simulink model "Solver_simulink"  (R2026a)
settings: Solver=VariableStepAuto  StopTime=5  RelTol=1e-4
values from neighbouring files (symbols this model uses):
  a = 0.01    [MassSpringDamper.m]    (also in Quarter_Car_Sim.m = 8; Simscape_Matlab.m = 8; Suspension_Sim.m = 8)
  c = 30000    [MassSpringDamper.m]    (also in Quarter_Car_Sim.m = c0 + c0*(0.005*(trialNum-1)); RoadSuite.m = 700; Simscape_Matlab.m = c0 + c0*(0.005*(trialNum-1)); Suspension_Sim.m = c0 + c0*(0.005*(trialNum-1)))
  Ks = Ks0 + Ks0*(0.005*(trialNum-1))    [Quarter_Car_Sim.m]    (also in RoadSuite.m = 30647.196473; Simscape_Matlab.m; Suspension_Sim.m)
  Kt = 114182.69772    [Quarter_Car_Sim.m]    (also in RoadSuite.m; Simscape_Matlab.m = 114182.6977; Suspension_Sim.m = 114182.6977)
  M = 108    [Quarter_Car_Sim.m]    (also in RoadSuite.m; Simscape_Matlab.m = 54.2237; Suspension_Sim.m = 54.2237)
  m = 2600    [MassSpringDamper.m]    (also in Quarter_Car_Sim.m = 50; RoadSuite.m = 50; Simscape_Matlab.m = 22.6796; Suspension_Sim.m = 22.6796)
  S = input('Which profile do you want to optimize for? ')    [Simscape_Matlab.m]    (also in Suspension_Sim.m)
  v = v*0.44704    [Simscape_Matlab.m]    (also in Suspension_Sim.m)
undefined symbols (not defined in the file or in its folder): X, Y, Z
libraries: sm_lib x9, nesl_utility x3, simulink x1
settings Model: Creator=achilles  LastModifiedBy=achilles

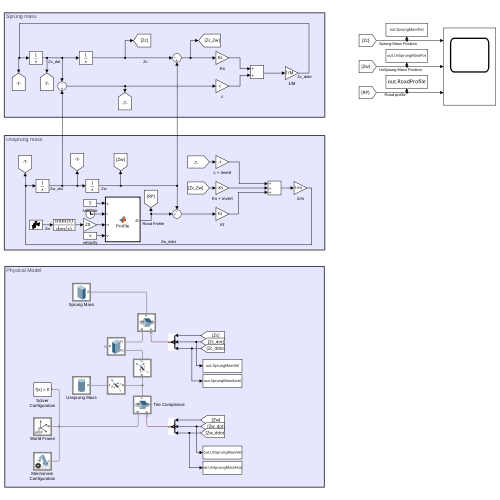
[thumbnail: Simulink's stored preview of the top-level diagram]
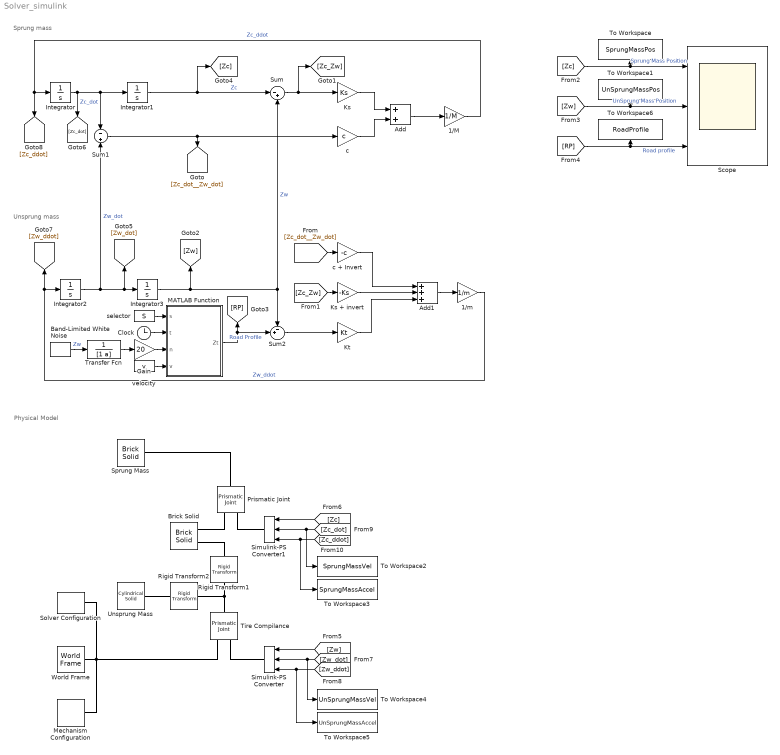
== system Solver_simulink ==
  note: Physical Model
  note: Unsprung mass
  note: Sprung mass
  1/M : Gain  Gain=1/M
  1/m : Gain  Gain=1/m
  Add : Sum
  Add1 : Sum  Inputs=+++
  Band-Limited White Noise : simulink/Sources/Band-Limited White Noise  Cov=[1e-7]  Ts=0.01  seed=[23331]
  Brick Solid : sm_lib/Body Elements/Brick Solid  BrickDimensions=[2 2 15]  BrickDimensionsUnits=in  ExportEntireGeometry=off  InertiaType=CalculateFromGeometry  BasedOnType=Density  Density=1000  DensityUnits=kg/m^3  Mass=1  MassUnits=kg  CenterOfMass=[0 0 0]  CenterOfMassUnits=m  MomentsOfInertia=[1 1 1]  MomentsOfInertiaUnits=kg*m^2  ProductsOfInertia=[0 0 0]  ProductsOfInertiaUnits=kg*m^2  GraphicType=FromGeometry  MarkerShape=Sphere  MarkerSize=10  GraphicVisPropType=SimpleVisualProperties  GraphicDiffuseColor=[0.5 0.5 0.5]  GraphicOpacity=1  GraphicSpecularColor=[0.5 0.5 0.5 1.0]  GraphicAmbientColor=[0.15 0.15 0.15 1.0]  GraphicEmissiveColor=[0.0 0.0 0.0 1.0]  GraphicShininess=75  DoExposeReferenceFrame=on  SerializedFrames=|
      | <Frames>
      | 
      |   <Frame>
      |     <Id>Frame1</Id>
      |     <Value>
      |       <Name>F1</Name>
      |       <Origin>
      |         <Source>GeometricFeature</Source>
      |         <FeatureName>+z surface</FeatureName>
      |       </Origin>
      |       <PrimaryAxis>
      |         <DefinedDirection>+Z</DefinedDirection>
      |         <Source>ReferenceFrame</Source>
      |         <SourceDirection>+Z</SourceDirection>
      |         <FeatureName></FeatureName>
      |       </PrimaryAxis>
      |       <SecondaryAxis>
      |         <DefinedDirection>+X</DefinedDirection>
      |         <Source>ReferenceFrame</Source>
      |         <SourceDirection>+X</SourceDirection>
      |         <FeatureName></FeatureName>
      |       </SecondaryAxis>
      |     </Value>
      |   </Frame>
      | 
      |   <Frame>
      |     <Id>Frame2</Id>
      |     <Value>
      |       <Name>F2</Name>
      |       <Origin>
      |         <Source>GeometricFeature</Source>
      |         <FeatureName>-z surface</FeatureName>
      |       </Origin>
      |       <PrimaryAxis>
      |         <DefinedDirection>+Z</DefinedDirection>
      |         <Source>ReferenceFrame</Source>
      |         <SourceDirection>+Z</SourceDirection>
      |         <FeatureName></FeatureName>
      |       </PrimaryAxis>
      |       <SecondaryAxis>
      |         <DefinedDirection>+X</DefinedDirection>
      |         <Source>ReferenceFrame</Source>
      |         <SourceDirection>+X</SourceDirection>
      |         <FeatureName></FeatureName>
      |       </SecondaryAxis>
      |     </Value>
      |   </Frame>
      | 
      | </Frames>
  Clock : Clock
  Gain : Gain  Gain=20
  Integrator{,1..3} (4 alike) : Integrator
  Ks : Gain  Gain=Ks
  Ks + invert : Gain  Gain=-Ks
  Kt : Gain  Gain=Kt
  MATLAB Function : MATLAB Function  TreatAsAtomicUnit=on
  Mechanism Configuration : sm_lib/Utilities/Mechanism Configuration  UniformGravity=Constant  GravityVector=[0 0 -9.80665]  GravityVectorUnits=m/s^2  LinearizationDelta=0.001  JointModeTransitionNonlinearIterations=2
  Prismatic Joint : sm_lib/Joints/Prismatic Joint  JointMode=Normal  CompositeWrenchDir=FollowerOnBase  CompositeWrenchFrame=BaseFrame  SenseConstraintForce=off  SenseConstraintTorque=off  SenseTotalForce=off  SenseTotalTorque=off  PositionTargetSpecify=off  PositionTargetPriority=High  PositionTargetValue=0  PositionTargetValueUnits=m  VelocityTargetSpecify=off  VelocityTargetPriority=High  VelocityTargetValue=0  VelocityTargetValueUnits=m/s  EquilibriumPosition=0  EquilibriumPositionUnits=m  SpringStiffness=0  SpringStiffnessUnits=N/m  DampingCoefficient=0  DampingCoefficientUnits=N/(m/s)  LowerLimitSpecify=off  LowerLimitBound=-1  LowerLimitBoundUnits=m  LowerLimitStiffness=1e6  LowerLimitStiffnessUnits=N/m  LowerLimitDamping=1e3  LowerLimitDampingUnits=N/(m/s)  LowerLimitTransitionRegionWidth=1e-4  LowerLimitTransitionRegionWidthUnits=m  UpperLimitSpecify=off  UpperLimitBound=1  UpperLimitBoundUnits=m  UpperLimitStiffness=1e6  UpperLimitStiffnessUnits=N/m  UpperLimitDamping=1e3  UpperLimitDampingUnits=N/(m/s)  UpperLimitTransitionRegionWidth=1e-4  UpperLimitTransitionRegionWidthUnits=m  TorqueActuationMode=ComputedTorque  MotionActuationMode=InputMotion  SensePosition=off  SenseVelocity=off  SenseAcceleration=off  SenseTorqueForce=off  SenseLowerLimitTorqueForce=off  SenseUpperLimitTorqueForce=off
  Rigid Transform1 : sm_lib/Frames and Transforms/Rigid Transform  RotationMethod=None  FollAlignAxisA=+X  BaseAlignAxisA=+Y  FollAlignAxisB=+Y  BaseAlignAxisB=+Z  RotationStandardAxis=+X  RotationAngle=90  RotationAngleUnits=deg  RotationArbitraryAxis=[0 0 1]  RotationSequenceAxes=FollowerAxes  RotationSequence=XYX  RotationSequenceAngles=[0 0 0]  RotationSequenceAnglesUnits=deg  RotationMatrix=[1 0 0;0 1 0;0 0 1]  Quaternion=[1 0 0 0]  TranslationMethod=StandardAxis  TranslationCartesianOffset=[0 0 0]  TranslationCartesianOffsetUnits=m  TranslationStandardAxis=+Y  TranslationStandardOffset=7.5/2+1  TranslationStandardOffsetUnits=in  TranslationROffset=0  TranslationROffsetUnits=m  TranslationThetaOffset=0  TranslationThetaOffsetUnits=deg  TranslationZOffset=0  TranslationZOffsetUnits=m
  Rigid Transform2 : sm_lib/Frames and Transforms/Rigid Transform  RotationMethod=StandardAxis  FollAlignAxisA=+X  BaseAlignAxisA=+Y  FollAlignAxisB=+Y  BaseAlignAxisB=+Z  RotationStandardAxis=+X  RotationAngle=90  RotationAngleUnits=deg  RotationArbitraryAxis=[0 0 1]  RotationSequenceAxes=FollowerAxes  RotationSequence=XYX  RotationSequenceAngles=[0 0 0]  RotationSequenceAnglesUnits=deg  RotationMatrix=[1 0 0;0 1 0;0 0 1]  Quaternion=[1 0 0 0]  TranslationMethod=None  TranslationCartesianOffset=[0 0 0]  TranslationCartesianOffsetUnits=m  TranslationStandardAxis=+Y  TranslationStandardOffset=11  TranslationStandardOffsetUnits=in  TranslationROffset=0  TranslationROffsetUnits=m  TranslationThetaOffset=0  TranslationThetaOffsetUnits=deg  TranslationZOffset=0  TranslationZOffsetUnits=m
  Scope : Scope  NumInputPorts=3
      settings: ActiveDisplayYMinimum=-0.00882861869744846  ActiveDisplayYMaximum=0.013003201828368532
  Simulink-PS Converter : nesl_utility/Simulink-PS Converter  PhysicalDomain=network_engine_domain  SubClassName=ps_input  LeftPortType=input  RightPortType=output  PseudoPeriodic=off  Frequencies=[]  NoiseDistribution=none  NoiseParameters=[]  Unit=m  AffineConversion=off  FilteringAndDerivatives=provide  SimscapeFilterOrder=1  InputFilterTimeConstant=0.001  UdotUserProvided=2
  Simulink-PS Converter1 : nesl_utility/Simulink-PS Converter  PhysicalDomain=network_engine_domain  SubClassName=ps_input  LeftPortType=input  RightPortType=output  PseudoPeriodic=off  Frequencies=[]  NoiseDistribution=none  NoiseParameters=[]  Unit=m  AffineConversion=off  FilteringAndDerivatives=provide  SimscapeFilterOrder=1  InputFilterTimeConstant=0.001  UdotUserProvided=2
  Solver Configuration : nesl_utility/Solver Configuration  PhysicalDomain=network_engine_domain  SubClassName=solver  LeftPortType=input  RightPortType=generic  Tones=[]  Harmonics=[]  SimulateNoise=off  Profile=off  UseLocalSampling=off  EnableSwitchedLinearOptims=on  FrequencyDomain=off  UseCCode=off  RelTol=0.001  AbsTol=1e-06  MinStep=1e-09  ToWorkspace=off  RevertToSquareIcSolve=off  NumHomotopyIterations=100  PhasorMode=off  PhasorModeNumHarmonics=1  ConsistencySolver=NEWTON_XTOL_AFTER_FTOL  CanonicalOrdering=UNORDERED  OptimizeIntermediates=UNOPTIMIZED  IndexReductionMethod=DerivativeReplacement  DoDC=off  ResidualTolerance=1e-09  ConsistencyTolSource=GLOBAL  ConsistencyAbsTol=0.001  ConsistencyRelTol=0.001  ConsistencyTolFactor=0.001  UseLocalSolver=off  LocalSolverChoice=NE_BACKWARD_EULER_ADVANCER  ResolveIndetEquations=on  FunctionEvalNumThread=1  LocalSolverSampleTime=0.001  DoFixedCost=off  MaxNonlinIter=3  MaxModeIter=2  ComputeImpulses=off  ImpulseIterations=2  LinearAlgebra=Sparse  LinearAlgebraNumThread=0  EquationFormulation=NE_TIME_EF  DelaysMemoryBudget=1024  AutomaticFiltering=on  FilteringTimeConstant=0.001  PartitionStorageMethod=AS_NEEDED  PartitionMemoryBudget=1024  PartitionMethod=FAST  MultibodyUseLocalSolver=off  MultibodyLocalSolverChoice=ODE1  MultibodyLocalSolverSampleTime=0.001
  Sprung Mass : sm_lib/Body Elements/Brick Solid  BrickDimensions=[ 20 10 5]  BrickDimensionsUnits=in  ExportEntireGeometry=off  InertiaType=Custom  BasedOnType=Density  Density=1000  DensityUnits=kg/m^3  Mass=108  MassUnits=kg  CenterOfMass=[0 0 0]  CenterOfMassUnits=m  MomentsOfInertia=[1 1 1]  MomentsOfInertiaUnits=kg*m^2  ProductsOfInertia=[0 0 0]  ProductsOfInertiaUnits=kg*m^2  GraphicType=FromGeometry  MarkerShape=Sphere  MarkerSize=10  GraphicVisPropType=SimpleVisualProperties  GraphicDiffuseColor=[0.5 0.5 0.5]  GraphicOpacity=1  GraphicSpecularColor=[0.5 0.5 0.5 1.0]  GraphicAmbientColor=[0.15 0.15 0.15 1.0]  GraphicEmissiveColor=[0.0 0.0 0.0 1.0]  GraphicShininess=75  DoExposeReferenceFrame=on  SerializedFrames=<Frames/>
  Sum : Sum  Inputs=|-+
  Sum1 : Sum  Inputs=-+
  Sum2 : Sum  Inputs=-+|
  Tire Compilance : sm_lib/Joints/Prismatic Joint  JointMode=Normal  CompositeWrenchDir=FollowerOnBase  CompositeWrenchFrame=BaseFrame  SenseConstraintForce=off  SenseConstraintTorque=off  SenseTotalForce=off  SenseTotalTorque=off  PositionTargetSpecify=off  PositionTargetPriority=High  PositionTargetValue=0  PositionTargetValueUnits=m  VelocityTargetSpecify=off  VelocityTargetPriority=High  VelocityTargetValue=0  VelocityTargetValueUnits=m/s  EquilibriumPosition=0  EquilibriumPositionUnits=m  SpringStiffness=4500  SpringStiffnessUnits=N/m  DampingCoefficient=1000  DampingCoefficientUnits=N/(m/s)  LowerLimitSpecify=off  LowerLimitBound=-1  LowerLimitBoundUnits=m  LowerLimitStiffness=1e6  LowerLimitStiffnessUnits=N/m  LowerLimitDamping=1e3  LowerLimitDampingUnits=N/(m/s)  LowerLimitTransitionRegionWidth=1e-4  LowerLimitTransitionRegionWidthUnits=m  UpperLimitSpecify=off  UpperLimitBound=1  UpperLimitBoundUnits=m  UpperLimitStiffness=1e6  UpperLimitStiffnessUnits=N/m  UpperLimitDamping=1e3  UpperLimitDampingUnits=N/(m/s)  UpperLimitTransitionRegionWidth=1e-4  UpperLimitTransitionRegionWidthUnits=m  TorqueActuationMode=ComputedTorque  MotionActuationMode=InputMotion  SensePosition=off  SenseVelocity=off  SenseAcceleration=off  SenseTorqueForce=off  SenseLowerLimitTorqueForce=off  SenseUpperLimitTorqueForce=off
  To Workspace : ToWorkspace  VariableName=SprungMassPos  SaveFormat=Timeseries  SampleTime=-1
  To Workspace1 : ToWorkspace  VariableName=UnSprungMassPos  SaveFormat=Timeseries  SampleTime=-1
  To Workspace2 : ToWorkspace  VariableName=SprungMassVel  SaveFormat=Timeseries  SampleTime=-1
  To Workspace3 : ToWorkspace  VariableName=SprungMassAccel  SaveFormat=Timeseries  SampleTime=-1
  To Workspace4 : ToWorkspace  VariableName=UnSprungMassVel  SaveFormat=Timeseries  SampleTime=-1
  To Workspace5 : ToWorkspace  VariableName=UnSprungMassAccel  SaveFormat=Timeseries  SampleTime=-1
  To Workspace6 : ToWorkspace  VariableName=RoadProfile  SaveFormat=Timeseries  SampleTime=-1
  Transfer Fcn : TransferFcn  Denominator=[1 a]
  Unsprung Mass : sm_lib/Body Elements/Cylindrical Solid  CylinderRadius=8  CylinderRadiusUnits=in  CylinderLength=7.5  CylinderLengthUnits=in  ExportEntireGeometry=off  InertiaType=Custom  BasedOnType=Density  Density=1000  DensityUnits=kg/m^3  Mass=50  MassUnits=kg  CenterOfMass=[0 0 0]  CenterOfMassUnits=m  MomentsOfInertia=[1 1 1]  MomentsOfInertiaUnits=kg*m^2  ProductsOfInertia=[0 0 0]  ProductsOfInertiaUnits=kg*m^2  GraphicType=FromGeometry  MarkerShape=Sphere  MarkerSize=10  GraphicVisPropType=SimpleVisualProperties  GraphicDiffuseColor=[0.5 0.5 0.5]  GraphicOpacity=1  GraphicSpecularColor=[0.5 0.5 0.5 1.0]  GraphicAmbientColor=[0.15 0.15 0.15 1.0]  GraphicEmissiveColor=[0.0 0.0 0.0 1.0]  GraphicShininess=75  DoExposeReferenceFrame=on  SerializedFrames=<Frames/>
  World Frame : sm_lib/Frames and Transforms/World Frame
  c : Gain  Gain=c
  c + Invert : Gain  Gain=-c
  selector : Constant  Value=S
  velocity : Constant  Value=v
  wires:
  Integrator1/1 -> [Zc], Sum/1  "Zc"
  Integrator/1 -> [Zc_dot], Sum1/1, Integrator1/1  "Zc_dot"
  Ks/1 -> Add/1
  Add/1 -> 1/M/1
  c/1 -> Add/2
  1/M/1 -> Integrator/1, [Zc_ddot]  "Zc_ddot"
  Integrator3/1 -> [Zw], Sum/2, Sum2/1  "Zw"
  Clock/1 -> MATLAB Function/2(t)
  Integrator2/1 -> Integrator3/1, [Zw_dot], Sum1/2  "Zw_dot"
  c + Invert/1 -> Add1/1
  MATLAB Function/1(Zt) -> Sum2/2, [RP]  "Road Profile"
  Sum2/1 -> Kt/1
  Ks + invert/1 -> Add1/2
  Kt/1 -> Add1/3
  Sum1/1 -> c/1, [Zc_dot__Zw_dot]
  selector/1 -> MATLAB Function/1(s)
  Sum/1 -> [Zc_Zw], Ks/1
  Add1/1 -> 1/m/1
  1/m/1 -> Integrator2/1, [Zw_ddot]  "Zw_ddot"
  [Zc_dot__Zw_dot] -> c + Invert/1
  [Zc_Zw] -> Ks + invert/1
  [RP] -> To Workspace6/1, Scope/3  "Road profile"
  [Zc] -> Scope/1, To Workspace/1  "Sprung Mass Position"
  [Zw] -> Scope/2, To Workspace1/1  "UnSprung Mass Position"
  [Zw_ddot] -> To Workspace5/1, Simulink-PS Converter/3
  [Zw_dot] -> To Workspace4/1, Simulink-PS Converter/2
  [Zc] -> Simulink-PS Converter1/1
  [Zw] -> Simulink-PS Converter/1
  [Zc_ddot] -> To Workspace3/1, Simulink-PS Converter1/3
  [Zc_dot] -> To Workspace2/1, Simulink-PS Converter1/2
  Band-Limited White Noise/1 -> Transfer Fcn/1  "Zw"
  Transfer Fcn/1 -> Gain/1
  Gain/1 -> MATLAB Function/3(n)
  velocity/1 -> MATLAB Function/4(v)
  connections:
  Simulink-PS Converter/RConn1 -- Tire Compilance/LConn2
  Rigid Transform2/RConn1 -- Unsprung Mass/RConn1
  Simulink-PS Converter1/RConn1 -- Prismatic Joint/LConn2
  Prismatic Joint/LConn1 -- Brick Solid/LConn1
  Rigid Transform1/RConn1 -- Brick Solid/LConn2
  Mechanism Configuration/RConn1 -- World Frame/RConn1 -- Tire Compilance/LConn1 -- Solver Configuration/RConn1
  Prismatic Joint/RConn1 -- Sprung Mass/RConn1
  Rigid Transform2/LConn1 -- Rigid Transform1/LConn1 -- Tire Compilance/RConn1

== matlab function Solver_simulink/MATLAB Function ==
  data: s input; Zt output; t input; n input; v input
function Zt = Profile(s, t, n, v)

Zt = 0;
% Physical feature dimensions
Len_bump = .5;      % speed bump length
Len_wash = .5;       % washboard wavelength
heig_bump = 0.01;   % bump height, m
t0 = 1;             % bump start time, s

% Deriving impulse timing from speed
tauB = Len_bump/(2*v);    % time cross the hump
tauW = Len_wash/v;
wW   = pi/tauW;
wB   = pi/tauB;      % angular freq for one raised bump

% Smooth "pothole" bump
if s == 1
    if t < 1
        Zt = 0;
    elseif t<= t0 + 2*tauB
        Zt = (heig_bump/2)*cos(wB*(t-t0)) - heig_bump/2;
    else 
        Zt=0;
    end

    % Rough terrain
elseif s == 2
    Zt = n;

    % Washboards
elseif s == 3
    if t > 0.5
        Zt = -(heig_bump/2)*cos(wW*(t-0.5)) + heig_bump/2;
    end

    % Rough terrain + speed bump
elseif s == 4
    Zt = n;
    if (t >= t0) && (t <= t0 + tauB)
        Zt = -(heig_bump/2)*cos(wB*(t-t0)) + heig_bump/2;
    end
end
end
